simulink model "SeanModel"  (R2014a)
settings: Solver=ode3  StartTime=0.0  StopTime=30  RelTol=1e-3
undefined symbols (not defined in the file or in its folder): dfilt, fdesignblkfcn, gcbh
libraries: Solver_SF x1, dsparch4 x1
settings Model: Creator=zierdt.1  LastModifiedBy=zierdt.1

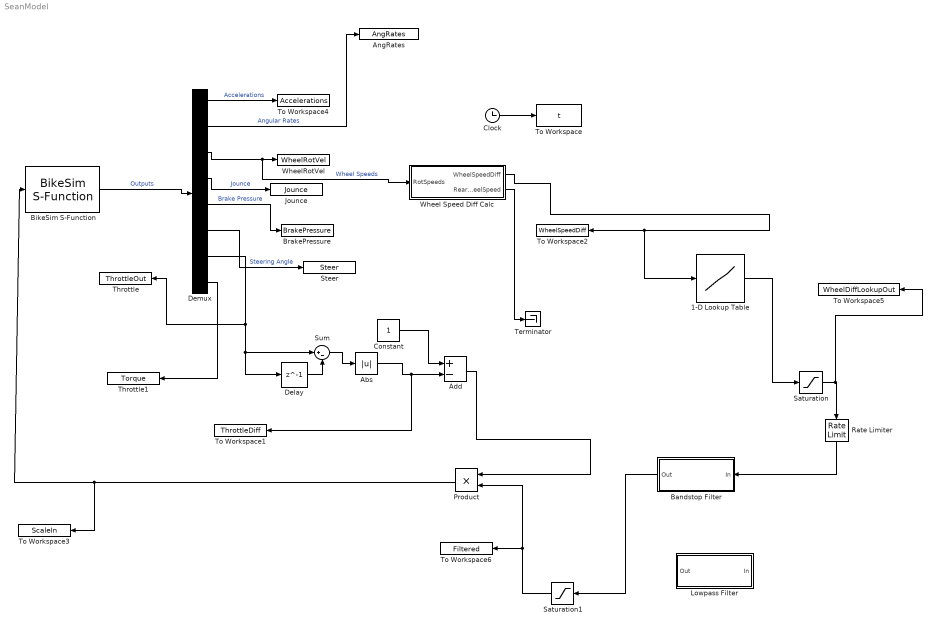
== system SeanModel ==
  1-D Lookup Table : Lookup_n-D  NumberOfTableDimensions=1  BreakpointsForDimension1=[3.5,4.5]  BreakpointsForDimension2=[0, 2 ,100,1000]  Table=[1,0]  InternalRulePriority=Speed  RndMeth=Simplest  InputSameDT=on
  Abs : Abs
  Add : Sum  Inputs=+-
  AngRates : ToWorkspace  VariableName=AngRates  SaveFormat=Timeseries  SampleTime=-1
  Bandstop Filter : Subsystem  DialogController=fdesignblkfcn  InitFcn=fdesignblkfcn(gcbh, {'InitFcn'});  mask(Bandstop Filter){}
      mask help: Design a bandstop filter
      settings: CopyFcn=fdesignblkfcn(gcbh, {'CopyFcn'});
      mask Help: helpview(mapfilelocation('dsp'), 'dspbandstopfilter');
      mask Display: disp('Bandstop');
  BikeSim S-Function : Solver_SF/BikeSim S-Function  Priority=1  VehicleCode=fixed_caster  SIMFILE=simfile.sim
      settings: AttributesFormatString=Vehicle Code: %<VehicleCode>
  BrakePressure : ToWorkspace  VariableName=BrakePressure  SaveFormat=Timeseries  SampleTime=-1
  Clock : Clock
  Constant : Constant
  Delay : Delay  DelayLength=1  InitialCondition=0
  Demux : Demux  Outputs=[3 2 2 2 2 1 1 3]
  Jounce : ToWorkspace  VariableName=Jounce  SaveFormat=Timeseries  SampleTime=-1
  Lowpass Filter : Subsystem  DialogController=fdesignblkfcn  InitFcn=fdesignblkfcn(gcbh, {'InitFcn'});  mask(Lowpass Filter){}
      mask help: Design a lowpass filter
      settings: CopyFcn=fdesignblkfcn(gcbh, {'CopyFcn'});
      mask Help: helpview(mapfilelocation('dsp'), 'dsplowpassfilter');
      mask Display: disp('Lowpass')
  Product : Product
  Rate Limiter : RateLimiter  RisingSlewLimit=200  FallingSlewLimit=-725  SampleTimeMode=inherited
  Saturation : Saturate  UpperLimit=1  LowerLimit=0
  Saturation1 : Saturate  UpperLimit=1  LowerLimit=0
  Steer : ToWorkspace  VariableName=Steer  SaveFormat=Timeseries  SampleTime=-1
  Sum : Sum  Inputs=|+-
  Terminator : Terminator
  Throttle : ToWorkspace  VariableName=ThrottleOut  SaveFormat=Timeseries  SampleTime=-1
  Throttle1 : ToWorkspace  VariableName=Torque  SaveFormat=Timeseries  SampleTime=-1
  To Workspace : ToWorkspace  VariableName=t  SampleTime=-1
  To Workspace1 : ToWorkspace  VariableName=ThrottleDiff  SaveFormat=Timeseries  SampleTime=-1
  To Workspace2 : ToWorkspace  VariableName=WheelSpeedDiff  SaveFormat=Timeseries  SampleTime=-1
  To Workspace3 : ToWorkspace  VariableName=ScaleIn  SaveFormat=Timeseries  SampleTime=-1
  To Workspace4 : ToWorkspace  VariableName=Accelerations  SaveFormat=Timeseries  SampleTime=-1
  To Workspace5 : ToWorkspace  VariableName=WheelDiffLookupOut  SaveFormat=Timeseries  SampleTime=-1
  To Workspace6 : ToWorkspace  VariableName=Filtered  SaveFormat=Timeseries  SampleTime=-1
  Wheel Speed Diff Calc : Subsystem
  WheelRotVel : ToWorkspace  VariableName=WheelRotVel  SaveFormat=Timeseries  SampleTime=-1
  wires:
  Demux/1 -> To Workspace4/1  "Accelerations"
  Demux/3 -> Wheel Speed Diff Calc/1(RotSpeeds), WheelRotVel/1  "Wheel Speeds"
  Demux/4 -> Jounce/1  "Jounce"
  Demux/5 -> BrakePressure/1  "Brake Pressure"
  Demux/6 -> Steer/1  "Steering Angle"
  BikeSim S-Function/1 -> Demux/1  "Outputs"
  Clock/1 -> To Workspace/1
  Demux/2 -> AngRates/1  "Angular Rates"
  Delay/1 -> Sum/2
  Constant/1 -> Add/1
  Demux/7 -> Sum/1, Delay/1, Throttle/1
  Sum/1 -> Abs/1
  Abs/1 -> To Workspace1/1, Add/2
  Add/1 -> Product/1
  Demux/8 -> Throttle1/1
  Wheel Speed Diff Calc/1(WheelSpeedDiff) -> 1-D Lookup Table/1, To Workspace2/1
  1-D Lookup Table/1 -> Saturation/1
  Saturation/1 -> Rate Limiter/1, To Workspace5/1
  Product/1 -> To Workspace3/1, BikeSim S-Function/1
  Saturation1/1 -> To Workspace6/1, Product/2
  Bandstop Filter/1(Out) -> Saturation1/1
  Rate Limiter/1 -> Bandstop Filter/1(In)
  Wheel Speed Diff Calc/2(RearWheelSpeed) -> Terminator/1

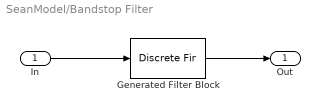
== system SeanModel/Bandstop Filter ==
  In : Inport
  Generated Filter Block : DiscreteFir  Tag=BlockMethodSubSystem  Coefficients=[-8.5482507973099828e-06 0.0028889633483420852 1.0814930644075384e-05 0.044841500985625955 -5.4668016452838353e-07 -0.013920546923225289 -1.2165002407744266e-05 -0.10727125660163835 2.071325320463912e-05 0.27257409150791967 -1.0268250479218759e-05 0.64877449009571175 -1.0268250479218759e-05 0.27257409150791967 2.071325320463912e-05 -0.10727125660163835 -1.2165002407744266e-05 -0.013920546923225289 -5.4668016452838353e-07 0.044841500985625955 1.0814930644075384e-05 0.0028889633483420852 -8.5482507973099828e-06]  InputProcessing=Columns as channels (frame based)
  Out : Outport
  wires:
  Generated Filter Block/1 -> Out/1
  In/1 -> Generated Filter Block/1

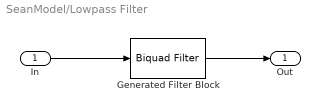
== system SeanModel/Lowpass Filter ==
  In : Inport
  Generated Filter Block : dsparch4/Biquad Filter  Tag=BlockMethodSubSystem  IIRFiltStruct=Direct form II  CoeffSource=Specify via dialog  BiQuadCoeffs=[0.35230146550854152 0.70460293101708305 0.35230146550854152 1 -0.18062861276293468 0.53038926211178405;0.37244578900933756 0.74489157801867512 0.37244578900933756 1 -0.13693336440674406 0.16017804326471285;0.29855268988135275 0.5971053797627055 0.29855268988135275 1 -0.12032531746022769 0.019465138909104326;0.47159705718998224 0.47159705718998224 0 1 -0.059220912888930811 0;0.28757913514155453 0.57515827028310906 0.28757913514155453 1 -0.12622078183180585 0.069414896211770119;0.12715010224927567 0.25430020449855134 0.12715010224927567 1 -0.15407520680966669 0.30541356904863526;0.25769180793642382 0.51538361587284764 0.25769180793642382 1 -0.22220117092993169 0.88261583155784673;0.38371715199711864 0.76743430399423729 0.38371715199711864 1 -0.16590894239324383 0.40567576777096676;0.4241945043675025 0.848389008735005 0.4241945043675025 1 -0.13089759638917958 0.10903955295918411;0.30073110142976406 0.60146220285952812 0.30073110142976406 1 -0.11890899806690422 0.007465268245713438;0.2700517711378963 0.5401035422757926 0.2700517711378963 1 -0.12273619539171698 0.039891480241060456;0.22383459775733791 0.44766919551467582 0.22383459775733791 1 -0.14455622726397821 0.2247633118155635;0.41526636234151509 0.83053272468303019 0.41526636234151509 1 -0.1990232141590243 0.6862388809888802]  a0Flag=Warning  IC=0  ICnum=0  ICden=0  InputProcessing=Columns as channels (frame based)  denAccumFracLength=30  denProdOutputFracLength=30  secondMemoryFracLength=15  roundingMode=Floor  overflowMode=off  ScaleValues=[0.46598578007750174;1;1;1;1;1;1;1;1;1;1;1;1;1]  optimizeScaleValues=off  ScaleValueMode=Specify via input port (g)  scaleValueFracLength=14  FilterSource=Specify via dialog  dfiltObjectName=dfilt.df2tsos([1 0.3 0.4],[1 0.1 0.2])
  Out : Outport
  wires:
  In/1 -> Generated Filter Block/1
  Generated Filter Block/1 -> Out/1

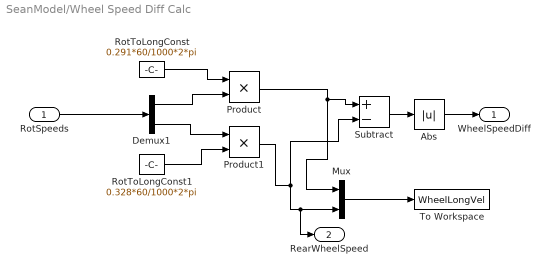
== system SeanModel/Wheel Speed Diff Calc ==
  RotSpeeds : Inport
  Abs : Abs
  Demux1 : Demux  Outputs=2
  Mux : Mux  Inputs=2
  Product : Product
  Product1 : Product
  RotToLongConst : Constant  Value=0.291*60/1000*2*pi
  RotToLongConst1 : Constant  Value=0.328*60/1000*2*pi
  Subtract : Sum  Inputs=+-
  To Workspace : ToWorkspace  VariableName=WheelLongVel  SaveFormat=Timeseries  SampleTime=-1
  WheelSpeedDiff : Outport
  RearWheelSpeed : Outport  Port=2
  wires:
  RotSpeeds/1 -> Demux1/1
  Demux1/1 -> Product/2
  Demux1/2 -> Product1/1
  RotToLongConst/1 -> Product/1
  RotToLongConst1/1 -> Product1/2
  Product/1 -> Subtract/1, Mux/1
  Product1/1 -> Subtract/2, RearWheelSpeed/1, Mux/2
  Subtract/1 -> Abs/1
  Abs/1 -> WheelSpeedDiff/1
  Mux/1 -> To Workspace/1
